simulink model "FrequencyModulation2"  (R2020b)
settings: Solver=VariableStepAuto  StartTime=0.0  StopTime=10  RelTol=1e-3
settings Model: Creator=Muthu  LastModifiedBy=Muthu

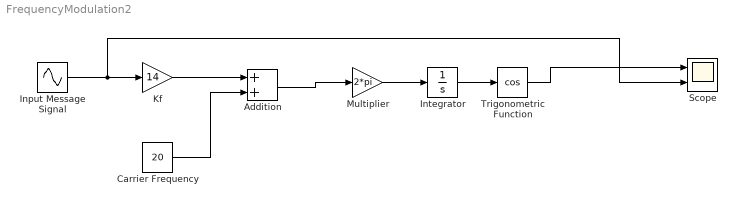
== system FrequencyModulation2 ==
  Addition : Sum
  Carrier Frequency : Constant  Value=20
  Input Message Signal : Sin  Frequency=2  SampleTime=0.001
  Integrator : Integrator
  Kf : Gain  Gain=14
  Multiplier : Gain  Gain=2*pi
  Scope : Scope  NumInputPorts=2
  Trigonometric Function : Trigonometry  Operator=cos
  wires:
  Input Message Signal/1 -> Scope/2, Kf/1
  Kf/1 -> Addition/1
  Carrier Frequency/1 -> Addition/2
  Addition/1 -> Multiplier/1
  Trigonometric Function/1 -> Scope/1
  Multiplier/1 -> Integrator/1
  Integrator/1 -> Trigonometric Function/1
